simulink library "mbd_s32k_examples"  (Simulink 9.0)
settings: Solver=FixedStepDiscrete  StartTime=0.0  StopTime=10.0  FixedStep=0.1  RelTol=1e-3  EnableMultiTasking=on
InitFcn:
  | mbd_s32k14_consistency_checks(bdroot(gcs));
(part 1 of 3)
settings Model: Creator=NXP MBDT Team  LastModifiedBy=nxa14941

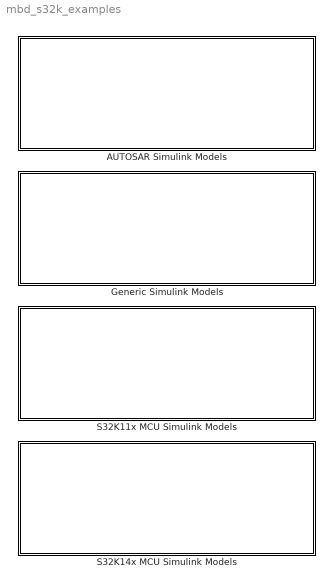
== system mbd_s32k_examples ==
  AUTOSAR Simulink Models : Subsystem
      mask Display: disp('AUTOSAR CLASSIC\n\nGenerate & Verify AUTOSAR Application Layer\non S32K1xx MCUs');
  Generic Simulink Models : Subsystem
      mask Display: disp('SIL - PIL - EXT MODE\n\nPROFILER - FREEMASTER - APPS\n\nGenerate & Verify Embedded Coder Code Generation\n on S32K1xx MCUs');
  S32K11x MCU Simulink Models : Subsystem
      mask Display: disp('S32K116, S32K118\nARM Cortex M0+\n\nCore, Systems, Peripherals, Utilities, AMMCLIB');
  S32K14x MCU Simulink Models : Subsystem
      mask Display: disp('S32K142, S32K144, S32K146, S32K148\nARM Cortex M4F\n\nCore, Systems, Peripherals, Utilities, AMMCLIB');

== system mbd_s32k_examples/AUTOSAR Simulink Models ==
  note: DISCLAIMER: All examples are distributed under the NXP Tools License Agreement Terms & Conditions
      | that can be found in LA_OPT_NXP_Software_License.htm
  note: AUTOSAR CLASSIC
      | Modelling, Verification and Validation
      | of Simulink Models on S32K1xx MCU
  "PIL " : Subsystem
      mask Display: disp('PIL\n(processor-in-the-loop)')

== system mbd_s32k_examples/Generic Simulink Models ==
  note: DISCLAIMER: All examples are distributed under the NXP Tools License Agreement Terms & Conditions that can be found in LA_OPT_NXP_Software_License.htm
  note: Modelling, Verification and Validation
      | of Simulink Models on S32K1xx MCU
  note: S32K1xx Applications
  External Mode : Subsystem
      mask Display: disp('EXTERNAL MODE')
  Miscellaneous Applications : Subsystem
      mask Display: disp('MISCELLANEOUS')
  "PIL " : Subsystem
      mask Display: disp('PIL\n(processor-in-the-loop)')
  SIL : Subsystem
      mask Display: disp('SIL\n(software-in-the-loop)')
  Utilities : Subsystem
      mask Display: disp('UTILITIES\nREGISTER ACCESS')

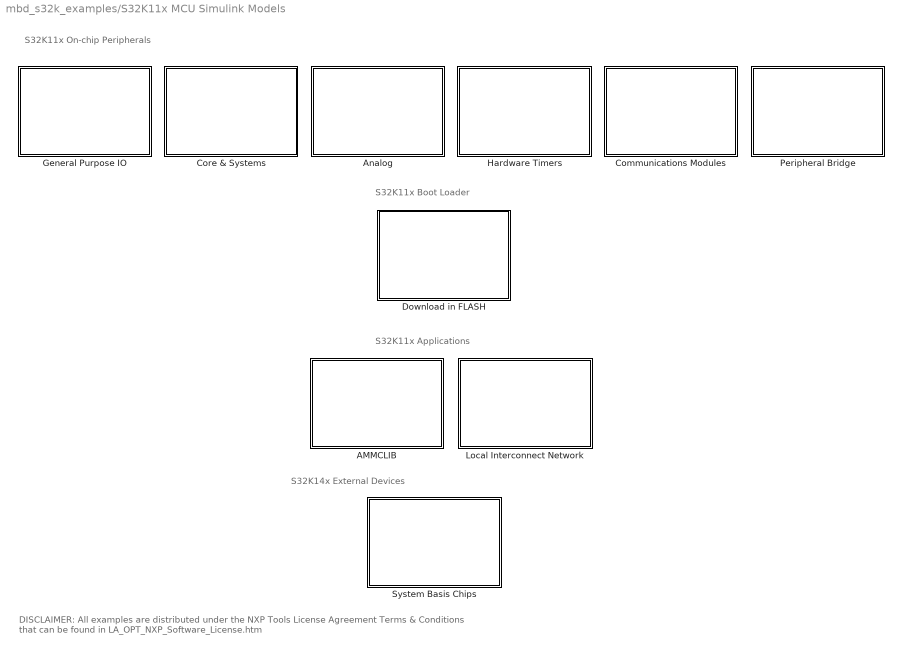
== system mbd_s32k_examples/S32K11x MCU Simulink Models ==
  note: S32K11x Boot Loader
  note: S32K11x On-chip Peripherals
  note: DISCLAIMER: All examples are distributed under the NXP Tools License Agreement Terms & Conditions that can be found in LA_OPT_NXP_Software_License.htm
  note: S32K11x Applications
  note: S32K14x External Devices
  AMMCLIB : Subsystem
      mask Display: disp('Automotive\nMath and Motor\nControl Library')
  Analog : Subsystem
      mask Display: disp('ADC\nCMP')
  Communications Modules : Subsystem
      mask Display: disp('UART\nSPI\nI2C\nFlexCAN\nFlexIO')
  Core & Systems : Subsystem
      mask Display: disp('PMC\nWDOG\nRTC\nEDMA\nLPTMR')
  Download in FLASH : Subsystem
      mask Display: disp('FLASH')
  General Purpose IO : Subsystem
      mask Display: disp('GPIO')
  Hardware Timers : Subsystem
      mask Display: disp('PDB\nFTM\nLPIT')
  Local Interconnect Network : Subsystem
      mask Display: disp('LIN')
  Peripheral Bridge : Subsystem
      mask Display: disp('MEMORIES\nREGISTERS')
  System Basis Chips : Subsystem
      mask Display: disp('SBC')

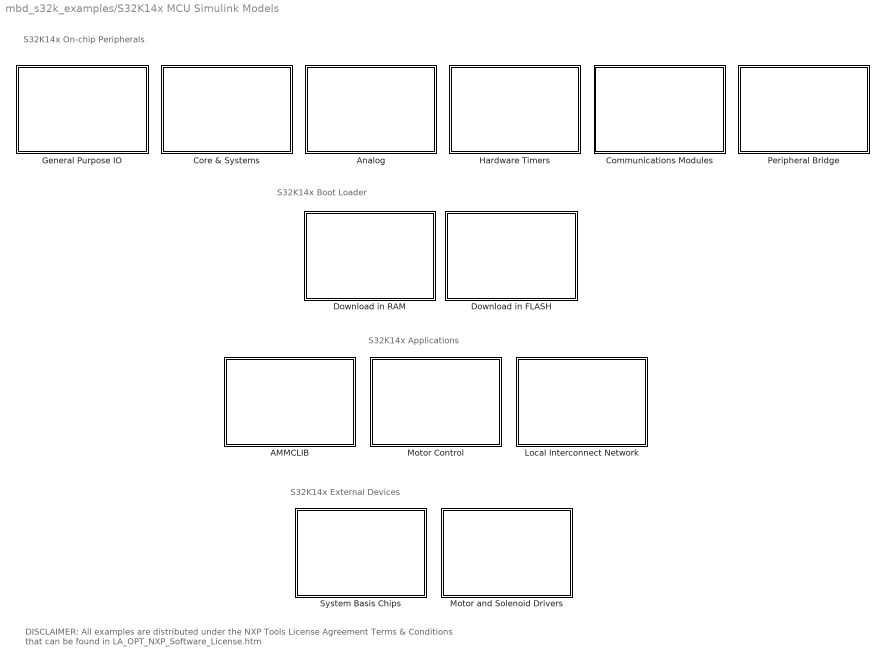
== system mbd_s32k_examples/S32K14x MCU Simulink Models ==
  note: S32K14x Boot Loader
  note: S32K14x External Devices
  note: DISCLAIMER: All examples are distributed under the NXP Tools License Agreement Terms & Conditions that can be found in LA_OPT_NXP_Software_License.htm
  note: S32K14x On-chip Peripherals
  note: S32K14x Applications
  AMMCLIB : Subsystem
      mask Display: disp('Automotive\nMath and Motor\nControl Library')
  Analog : Subsystem
      mask Display: disp('ADC\nCMP')
  Communications Modules : Subsystem
      mask Display: disp('UART\nSPI\nI2C\nFlexCAN\nFlexIO')
  Core & Systems : Subsystem
      mask Display: disp('PMC\nCSEC\nWDOG\nRTC\nEDMA\nLPTMR')
  Download in FLASH : Subsystem
      mask Display: disp('FLASH')
  Download in RAM : Subsystem
      mask Display: disp('RAM')
  General Purpose IO : Subsystem
      mask Display: disp('GPIO')
  Hardware Timers : Subsystem
      mask Display: disp('PDB\nFTM\nLPIT')
  Local Interconnect Network : Subsystem
      mask Display: disp('LIN')
  Motor Control : Subsystem
      mask Display: disp('MC')
  Motor and Solenoid Drivers : Subsystem
      mask Display: disp('TPP')
  Peripheral Bridge : Subsystem
      mask Display: disp('MEMORIES\nREGISTERS')
  System Basis Chips : Subsystem
      mask Display: disp('SBC')

== system mbd_s32k_examples/AUTOSAR Simulink Models/PIL  ==
  note: Note: PIL examples need a S32K1xx EVB to execute part of the generated code and a UART connection for getting the data out of the target. Make sure the UART port is configured correctly
  PIL_AS_Intergrator : Subsystem  mask{A=[]}
      mask prompts: A "Needed to invoke OpenFcn from the browser:"
      settings: OpenFcn=sfundemo_open('autosar_integrator_top_PIL')
      mask Display: disp('AUTOSAR PIL\nSimple Integrator');
  PIL_AS_Multiple_Runnables : Subsystem  mask{A=[]}
      mask prompts: A "Needed to invoke OpenFcn from the browser:"
      settings: OpenFcn=sfundemo_open('autosar_multirunnables_top_PIL')
      mask Display: disp('AUTOSAR PIL\nMultiple Runnables');
  PIL_AS_Throttle_Control : Subsystem  mask{A=[]}
      mask prompts: A "Needed to invoke OpenFcn from the browser:"
      settings: OpenFcn=sfundemo_open('mbdt_autosar_system_top')
      mask Display: disp('AUTOSAR PIL\nThrottle Control Example');

== system mbd_s32k_examples/Generic Simulink Models/External Mode ==
  External_Mode : Subsystem  mask{A=[]}
      mask prompts: A "Needed to invoke OpenFcn from the browser:"
      settings: OpenFcn=sfundemo_open('extmode_s32k1xx')
      mask Display: disp('EXTERNAL MODE\n Control Gauge in Simulink');

== system mbd_s32k_examples/Generic Simulink Models/Miscellaneous Applications ==
  Incremental Encoder : Subsystem  mask{A=[]}
      mask prompts: A "Needed to invoke OpenFcn from the browser:"
      settings: OpenFcn=sfundemo_open('ftm_incremental_encoder_s32k1xx')
      mask Display: disp('Incremental Encoder');

== system mbd_s32k_examples/Generic Simulink Models/PIL  ==
  note: Note: PIL examples need a S32K1xx EVB to execute part of the generated code and a UART connection for getting the data out of the target. Make sure the UART port is configured correctly
  PIL_AMMCLIB : Subsystem  mask{A=[]}
      mask prompts: A "Needed to invoke OpenFcn from the browser:"
      settings: OpenFcn=sfundemo_open('sim_pil_top_AMMCLIB_s32k1xx')
      mask Display: disp('AMMCLIB\n Sinusoidal signal generation');
  PIL_BLDC_Logic_Sequence : Subsystem  mask{A=[]}
      mask prompts: A "Needed to invoke OpenFcn from the browser:"
      settings: OpenFcn=sfundemo_open('sim_pil_top_BLDC_Commutation_s32k1xx')
      mask Display: disp('BLDC COMMUTATION\n Trapezoidal sequence commands\nand\nPWM signals output');
  PIL_RT_IO_STREAM : Subsystem  mask{A=[]}
      mask prompts: A "Needed to invoke OpenFcn from the browser:"
      settings: OpenFcn=sfundemo_open('mbd_s32k_rtiostreamtest')
      mask Display: disp('PIL TEST\nRT IO STREAM TEST');

== system mbd_s32k_examples/Generic Simulink Models/SIL ==
  SIL_AMMCLIB : Subsystem  mask{A=[]}
      mask prompts: A "Needed to invoke OpenFcn from the browser:"
      settings: OpenFcn=sfundemo_open('sim_sil_top_AMMCLIB_s32k1xx')
      mask Display: disp('AMMCLIB\n Sinusoidal signal generation');
  SIL_BLDC_Logic_Sequence : Subsystem  mask{A=[]}
      mask prompts: A "Needed to invoke OpenFcn from the browser:"
      settings: OpenFcn=sfundemo_open('sim_sil_top_BLDC_Commutation_s32k1xx')
      mask Display: disp('BLDC COMMUTATION\n Trapezoidal sequence commands\nand\nPWM signals output');
  SIL_Trapezoidal_Commutation : Subsystem  mask{A=[]}
      mask prompts: A "Needed to invoke OpenFcn from the browser:"
      settings: OpenFcn=sfundemo_open('sim_sil_top_TrapezoidalCommutation_s32k1xx')
      mask Display: disp('Trapezoidal\nCommutation');

== system mbd_s32k_examples/Generic Simulink Models/Utilities ==
  Custom_Initialization : Subsystem  mask{A=[]}
      mask prompts: A "Needed to invoke OpenFcn from the browser:"
      settings: OpenFcn=sfundemo_open('custom_init_s32k1xx')
      mask Display: disp('Custom Initialization\nCall custom code before\nat Simulink Initialize Fct');
  FreeMASTER_ISR_over_CAN : Subsystem  mask{A=[]}
      mask prompts: A "Needed to invoke OpenFcn from the browser:"
      settings: OpenFcn=sfundemo_open('fm_can_s32k1xx')
      mask Display: disp('FreeMASTER\n Data Visualization\nOver CAN');
  FreeMaster_ISR_over_UART : Subsystem  mask{A=[]}
      mask prompts: A "Needed to invoke OpenFcn from the browser:"
      settings: OpenFcn=sfundemo_open('fm_s32k1xx')
      mask Display: disp('FreeMASTER\nRECORDER and SCOPE\nInterrupt Based\nOver UART');
  FreeMaster_Polling_over_UART : Subsystem  mask{A=[]}
      mask prompts: A "Needed to invoke OpenFcn from the browser:"
      settings: OpenFcn=sfundemo_open('fm_polling_s32k1xx')
      mask Display: disp('FreeMASTER\n Polling Based\nOver UART');
  Profile_Application : Subsystem  mask{A=[]}
      mask prompts: A "Needed to invoke OpenFcn from the browser:"
      settings: OpenFcn=sfundemo_open('profiler_s32k1xx')
      mask Display: disp('PROFILER\nMeasure \nExecution Cycles');

== system mbd_s32k_examples/S32K11x MCU Simulink Models/AMMCLIB ==
  AMCLIB : Subsystem
      mask Display: disp('Advanced Motor Control Library\n\nBackEMF Observer,\n Tracking Observer,\n Speed and Current Loops');
  GDFLIB : Subsystem
      mask Display: disp('General Digital Filters Library\n\nFIR, IIR1, IIR2, Moving Average');
  GFLIB : Subsystem
      mask Display: disp('General Function Library\n\nSIN, ASIN, COS, ACOS, TAN, ATAN,\nLUT, LOG, Ramp, Hysteresis, Limit,\nPIp and PIr controllers');
  GMCLIB : Subsystem
      mask Display: disp('General Motor Control Library\n\nPark/Clark Direct&Inverse transformations,\n Space Vector Modulation,\n PMSM Decoupling,\n DC Bus Ripple Elimination');
  MLIB : Subsystem
      mask Display: disp('Mathematical Library\n\nABS, ADD, SUB, DIV, MUL, MAC,\nShifting, F16/F32/FLT Conversion');

== system mbd_s32k_examples/S32K11x MCU Simulink Models/Analog ==
  ADC_Potentiometer : Subsystem  mask{A=[]}
      mask prompts: A "Needed to invoke OpenFcn from the browser:"
      settings: OpenFcn=sfundemo_open('adc_software_trigger_s32k11x')
      mask Display: disp('ADC\nRead values from\npotentiometer');
  ADC_Software_Triggered : Subsystem  mask{A=[]}
      mask prompts: A "Needed to invoke OpenFcn from the browser:"
      settings: OpenFcn=sfundemo_open('adc_isr_s32k11x')
      mask Display: disp('ADC\nISR');
  CMP_IO_Triggering : Subsystem  mask{A=[]}
      mask prompts: A "Needed to invoke OpenFcn from the browser:"
      settings: OpenFcn=sfundemo_open('cmp_s32k11x')
      mask Display: disp('CMP\nCompare signals');
  FTM_PDB_ADC_Sync_Chaining : Subsystem  mask{A=[]}
      mask prompts: A "Needed to invoke OpenFcn from the browser:"
      settings: OpenFcn=sfundemo_open('ftm_pdb_adc_chaining_s32k11x')
      mask Display: disp('FTM-PDB-ADC\nChaining');

== system mbd_s32k_examples/S32K11x MCU Simulink Models/Communications Modules ==
  CAN : Subsystem
      mask Display: disp('FlexCAN')
  FlexIO : Subsystem
      mask Display: disp('FlexIO')
  I2C : Subsystem
      mask Display: disp('I2C')
  SPI : Subsystem
      mask Display: disp('SPI')
  Serial : Subsystem
      mask Display: disp('UART')

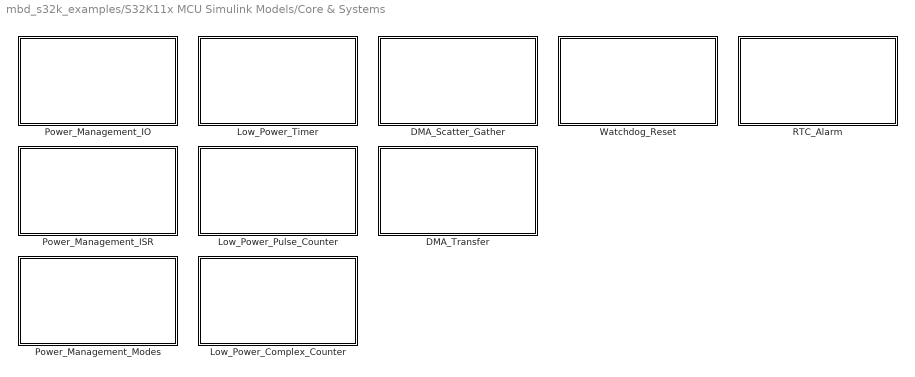
== system mbd_s32k_examples/S32K11x MCU Simulink Models/Core & Systems ==
  DMA_Scatter_Gather : Subsystem  mask{A=[]}
      mask prompts: A "Needed to invoke OpenFcn from the browser:"
      settings: OpenFcn=sfundemo_open('edma_scatter_gather_transfer_s32k11x')
      mask Display: disp('EDMA\n Scatter Gather Transfer');
  DMA_Transfer : Subsystem  mask{A=[]}
      mask prompts: A "Needed to invoke OpenFcn from the browser:"
      settings: OpenFcn=sfundemo_open('edma_simple_single_block_transfer_s32k11x')
      mask Display: disp('EDMA\n Simple Single Transfer');
  Low_Power_Complex_Counter : Subsystem  mask{A=[]}
      mask prompts: A "Needed to invoke OpenFcn from the browser:"
      settings: OpenFcn=sfundemo_open('lptmr_complex_time_counter_s32k11x')
      mask Display: disp('LPTMR\n Complex Time Counter');
  Low_Power_Pulse_Counter : Subsystem  mask{A=[]}
      mask prompts: A "Needed to invoke OpenFcn from the browser:"
      settings: OpenFcn=sfundemo_open('lptmr_pulse_counter_s32k11x')
      mask Display: disp('LPTMR\n Pulse Counter');
  Low_Power_Timer : Subsystem  mask{A=[]}
      mask prompts: A "Needed to invoke OpenFcn from the browser:"
      settings: OpenFcn=sfundemo_open('lptmr_time_counter_s32k11x')
      mask Display: disp('LPTMR\n Time Counter');
  Power_Management_IO : Subsystem  mask{A=[]}
      mask prompts: A "Needed to invoke OpenFcn from the browser:"
      settings: OpenFcn=sfundemo_open('pmc_gpio_s32k11x')
      mask Display: disp('PMC\nPower modes via GPIO');
  Power_Management_ISR : Subsystem  mask{A=[]}
      mask prompts: A "Needed to invoke OpenFcn from the browser:"
      settings: OpenFcn=sfundemo_open('pmc_callbacks_s32k11x')
      mask Display: disp('PMC\nPower modes Callbacks\n via GPIO');
  Power_Management_Modes : Subsystem  mask{A=[]}
      mask prompts: A "Needed to invoke OpenFcn from the browser:"
      settings: OpenFcn=sfundemo_open('pmc_vlpr_s32k11x')
      mask Display: disp('PMC\n Example Very Low Power Run');
  RTC_Alarm : Subsystem  mask{A=[]}
      mask prompts: A "Needed to invoke OpenFcn from the browser:"
      settings: OpenFcn=sfundemo_open('rtc_s32k11x')
      mask Display: disp('RTC');
  Watchdog_Reset : Subsystem  mask{A=[]}
      mask prompts: A "Needed to invoke OpenFcn from the browser:"
      settings: OpenFcn=sfundemo_open('wdog_s32k11x')
      mask Display: disp('WDOG');

== system mbd_s32k_examples/S32K11x MCU Simulink Models/Download in FLASH ==
  FLASH_BAM_S32K116 : Subsystem  mask{A=[]}
      mask prompts: A "Needed to invoke OpenFcn from the browser:"
      settings: OpenFcn=sfundemo_open('flash_bam_download_s32k116')
      mask Display: disp('S32K116\nDownload in Flash');
  FLASH_BAM_S32K118 : Subsystem  mask{A=[]}
      mask prompts: A "Needed to invoke OpenFcn from the browser:"
      settings: OpenFcn=sfundemo_open('flash_bam_download_s32k118')
      mask Display: disp('S32K118\nDownload in Flash');

== system mbd_s32k_examples/S32K11x MCU Simulink Models/General Purpose IO ==
  GPIO_ISR : Subsystem  mask{A=[]}
      mask prompts: A "Needed to invoke OpenFcn from the browser:"
      settings: OpenFcn=sfundemo_open('gpio_isr_control_s32k11x')
      mask Display: disp('GPIO\nISR Control');
  GPIO_S32K11xEVB : Subsystem  mask{A=[]}
      mask prompts: A "Needed to invoke OpenFcn from the browser:"
      settings: OpenFcn=sfundemo_open('gpio_s32k11x')
      mask Display: disp('GPIO on S32K11x\nLED & Buttons');

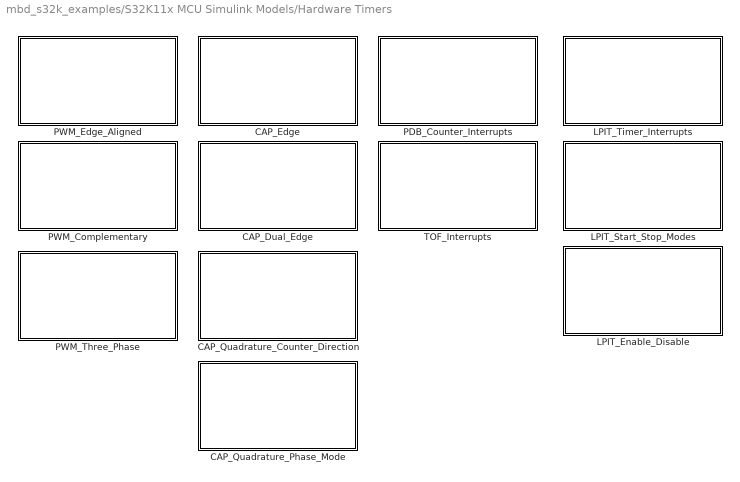
== system mbd_s32k_examples/S32K11x MCU Simulink Models/Hardware Timers ==
  CAP_Dual_Edge : Subsystem  mask{A=[]}
      mask prompts: A "Needed to invoke OpenFcn from the browser:"
      settings: OpenFcn=sfundemo_open('ftm_dual_edge_s32k11x')
      mask Display: disp('FTM\nDual Edge-Capture');
  CAP_Edge : Subsystem  mask{A=[]}
      mask prompts: A "Needed to invoke OpenFcn from the browser:"
      settings: OpenFcn=sfundemo_open('ftm_input_capture_s32k11x')
      mask Display: disp('FTM\nEdge-Capture');
  CAP_Quadrature_Counter_Direction : Subsystem  mask{A=[]}
      mask prompts: A "Needed to invoke OpenFcn from the browser:"
      settings: OpenFcn=sfundemo_open('ftm_qd_counter_s32k11x')
      mask Display: disp('FTM\nQuadrature-Capture\nCounter & Direction');
  CAP_Quadrature_Phase_Mode : Subsystem  mask{A=[]}
      mask prompts: A "Needed to invoke OpenFcn from the browser:"
      settings: OpenFcn=sfundemo_open('ftm_qd_phase_s32k11x')
      mask Display: disp('FTM\nQuadrature-Capture\nPhase Mode');
  LPIT_Enable_Disable : Subsystem  mask{A=[]}
      mask prompts: A "Needed to invoke OpenFcn from the browser:"
      settings: OpenFcn=sfundemo_open('lpit_s32k11x_enable_disable')
      mask Display: disp('LPIT\nEnable Disable');
  LPIT_Start_Stop_Modes : Subsystem  mask{A=[]}
      mask prompts: A "Needed to invoke OpenFcn from the browser:"
      settings: OpenFcn=sfundemo_open('lpit_s32k11x_start_stop')
      mask Display: disp('LPIT\nStart Stop');
  LPIT_Timer_Interrupts : Subsystem  mask{A=[]}
      mask prompts: A "Needed to invoke OpenFcn from the browser:"
      settings: OpenFcn=sfundemo_open('lpit_s32k11x')
      mask Display: disp('LPIT\nTimer interrupts');
  PDB_Counter_Interrupts : Subsystem  mask{A=[]}
      mask prompts: A "Needed to invoke OpenFcn from the browser:"
      settings: OpenFcn=sfundemo_open('pdb_s32k11x')
      mask Display: disp('PDB\nTimer interrupts');
  PWM_Complementary : Subsystem  mask{A=[]}
      mask prompts: A "Needed to invoke OpenFcn from the browser:"
      settings: OpenFcn=sfundemo_open('ftm_complementary_pwm_s32k11x')
      mask Display: disp('FTM\nComplementary\nPWM generation');
  PWM_Edge_Aligned : Subsystem  mask{A=[]}
      mask prompts: A "Needed to invoke OpenFcn from the browser:"
      settings: OpenFcn=sfundemo_open('ftm_independent_pwm_s32k11x')
      mask Display: disp('FTM\nEdge-Aligned vs\nCenter-Aligned\nPWM generation');
  PWM_Three_Phase : Subsystem  mask{A=[]}
      mask prompts: A "Needed to invoke OpenFcn from the browser:"
      settings: OpenFcn=sfundemo_open('ftm_three_phase_pwm_s32k11x')
      mask Display: disp('FTM\n3-Phase\nPWM generation\nCobine Mode');
  TOF_Interrupts : Subsystem  mask{A=[]}
      mask prompts: A "Needed to invoke OpenFcn from the browser:"
      settings: OpenFcn=sfundemo_open('ftm_tof_s32k11x')
      mask Display: disp('TOF\nTimer Overflow');

== system mbd_s32k_examples/S32K11x MCU Simulink Models/Local Interconnect Network ==
  "LIN Master " : Subsystem  mask{A=[]}
      mask prompts: A "Needed to invoke OpenFcn from the browser:"
      settings: OpenFcn=sfundemo_open('lin_master_s32k11x')
      mask Display: disp('LIN MASTER');
  LIN Slave : Subsystem  mask{A=[]}
      mask prompts: A "Needed to invoke OpenFcn from the browser:"
      settings: OpenFcn=sfundemo_open('lin_slave_s32k11x')
      mask Display: disp('LIN Slave');

== system mbd_s32k_examples/S32K11x MCU Simulink Models/Peripheral Bridge ==
  Memory_Access_RW : Subsystem  mask{A=[]}
      mask prompts: A "Needed to invoke OpenFcn from the browser:"
      settings: OpenFcn=sfundemo_open('memory_s32k11x')
      mask Display: disp('MEMORY');
  Register_Access_RW : Subsystem  mask{A=[]}
      mask prompts: A "Needed to invoke OpenFcn from the browser:"
      settings: OpenFcn=sfundemo_open('rw_registers_s32k11x')
      mask Display: disp('REGISTER');

== system mbd_s32k_examples/S32K11x MCU Simulink Models/System Basis Chips ==
  SBC_RW_Registers : Subsystem  mask{A=[]}
      mask prompts: A "Needed to invoke OpenFcn from the browser:"
      settings: OpenFcn=sfundemo_open('sbc_uja1169_rw_reg_s32k11x')
      mask Display: disp('UJA 1169\nRead/Write Registers');
  UJA1169_Control : Subsystem  mask{A=[]}
      mask prompts: A "Needed to invoke OpenFcn from the browser:"
      settings: OpenFcn=sfundemo_open('sbc_uja1169_mode_control_s32k11x')
      mask Display: disp('UJA 1169\nControl Modes');

== system mbd_s32k_examples/S32K14x MCU Simulink Models/AMMCLIB ==
  AMCLIB : Subsystem
      mask Display: disp('Advanced Motor Control Library\n\nBackEMF Observer,\n Tracking Observer,\n Speed and Current Loops');
  GDFLIB : Subsystem
      mask Display: disp('General Digital Filters Library\n\nFIR, IIR1, IIR2, Moving Average');
  GFLIB : Subsystem
      mask Display: disp('General Function Library\n\nSIN, ASIN, COS, ACOS, TAN, ATAN,\nLUT, LOG, Ramp, Hysteresis, Limit,\nPIp and PIr controllers');
  GMCLIB : Subsystem
      mask Display: disp('General Motor Control Library\n\nPark/Clark Direct&Inverse transformations,\n Space Vector Modulation,\n PMSM Decoupling,\n DC Bus Ripple Elimination');
  MLIB : Subsystem
      mask Display: disp('Mathematical Library\n\nABS, ADD, SUB, DIV, MUL, MAC,\nShifting, F16/F32/FLT Conversion');

== system mbd_s32k_examples/S32K14x MCU Simulink Models/Analog ==
  ADC_Hardware_Triggered : Subsystem  mask{A=[]}
      mask prompts: A "Needed to invoke OpenFcn from the browser:"
      settings: OpenFcn=sfundemo_open('adc_pdb_trigger_s32k14x')
      mask Display: disp('ADC\nConversion based on\nharware interrupts');
  ADC_Potentiometer : Subsystem  mask{A=[]}
      mask prompts: A "Needed to invoke OpenFcn from the browser:"
      settings: OpenFcn=sfundemo_open('adc_software_trigger_s32k14x')
      mask Display: disp('ADC\nRead values from\npotentiometer');
  ADC_Software_Triggered : Subsystem  mask{A=[]}
      mask prompts: A "Needed to invoke OpenFcn from the browser:"
      settings: OpenFcn=sfundemo_open('adc_isr_s32k14x')
      mask Display: disp('ADC\nISR');
  CMP_IO_Triggering : Subsystem  mask{A=[]}
      mask prompts: A "Needed to invoke OpenFcn from the browser:"
      settings: OpenFcn=sfundemo_open('cmp_s32k14x')
      mask Display: disp('CMP\nCompare signals');
  FTM_PDB_ADC_Sync_Chaining : Subsystem  mask{A=[]}
      mask prompts: A "Needed to invoke OpenFcn from the browser:"
      settings: OpenFcn=sfundemo_open('ftm_pdb_adc_chaining_s32k14x')
      mask Display: disp('FTM-PDB-ADC\nChaining');

== system mbd_s32k_examples/S32K14x MCU Simulink Models/Communications Modules ==
  CAN : Subsystem
      mask Display: disp('FlexCAN')
  FlexIO : Subsystem
      mask Display: disp('FlexIO')
  I2C : Subsystem
      mask Display: disp('I2C')
  SPI : Subsystem
      mask Display: disp('SPI')
  Serial : Subsystem
      mask Display: disp('UART')

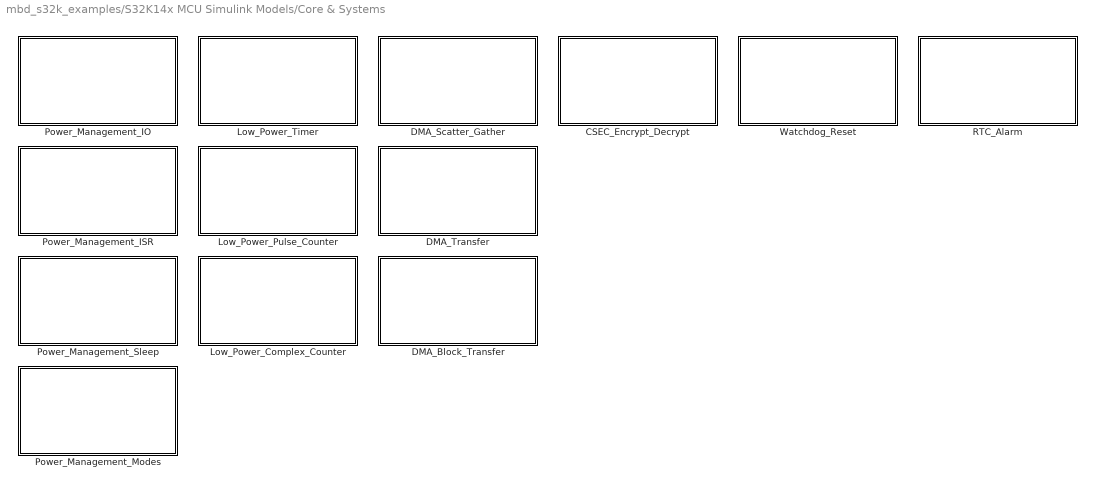
== system mbd_s32k_examples/S32K14x MCU Simulink Models/Core & Systems ==
  CSEC_Encrypt_Decrypt : Subsystem  mask{A=[]}
      mask prompts: A "Needed to invoke OpenFcn from the browser:"
      settings: OpenFcn=sfundemo_open('csec_keyconfig_s32k14x')
      mask Display: disp('CSEC');
  DMA_Block_Transfer : Subsystem  mask{A=[]}
      mask prompts: A "Needed to invoke OpenFcn from the browser:"
      settings: OpenFcn=sfundemo_open('edma_single_block_transfer_profiling_s32k14x')
      mask Display: disp('EDMA\n Single Block Transfer Profiling');
  DMA_Scatter_Gather : Subsystem  mask{A=[]}
      mask prompts: A "Needed to invoke OpenFcn from the browser:"
      settings: OpenFcn=sfundemo_open('edma_scatter_gather_transfer_s32k14x')
      mask Display: disp('EDMA\n Scatter Gather Transfer');
  DMA_Transfer : Subsystem  mask{A=[]}
      mask prompts: A "Needed to invoke OpenFcn from the browser:"
      settings: OpenFcn=sfundemo_open('edma_simple_single_block_transfer_s32k14x')
      mask Display: disp('EDMA\n Simple Single Transfer');
  Low_Power_Complex_Counter : Subsystem  mask{A=[]}
      mask prompts: A "Needed to invoke OpenFcn from the browser:"
      settings: OpenFcn=sfundemo_open('lptmr_complex_time_counter_s32k14x')
      mask Display: disp('LPTMR\n Complex Time Counter');
  Low_Power_Pulse_Counter : Subsystem  mask{A=[]}
      mask prompts: A "Needed to invoke OpenFcn from the browser:"
      settings: OpenFcn=sfundemo_open('lptmr_pulse_counter_s32k14x')
      mask Display: disp('LPTMR\n Pulse Counter');
  Low_Power_Timer : Subsystem  mask{A=[]}
      mask prompts: A "Needed to invoke OpenFcn from the browser:"
      settings: OpenFcn=sfundemo_open('lptmr_time_counter_s32k14x')
      mask Display: disp('LPTMR\n Time Counter');
  Power_Management_IO : Subsystem  mask{A=[]}
      mask prompts: A "Needed to invoke OpenFcn from the browser:"
      settings: OpenFcn=sfundemo_open('pmc_gpio_s32k14x')
      mask Display: disp('PMC\nPower modes via GPIO');
  Power_Management_ISR : Subsystem  mask{A=[]}
      mask prompts: A "Needed to invoke OpenFcn from the browser:"
      settings: OpenFcn=sfundemo_open('pmc_callbacks_s32k14x')
      mask Display: disp('PMC\nPower modes Callbacks\n via GPIO');
  Power_Management_Modes : Subsystem  mask{A=[]}
      mask prompts: A "Needed to invoke OpenFcn from the browser:"
      settings: OpenFcn=sfundemo_open('pmc_vlpr_s32k14x')
      mask Display: disp('PMC\n Example Very Low Power Run');
  Power_Management_Sleep : Subsystem  mask{A=[]}
      mask prompts: A "Needed to invoke OpenFcn from the browser:"
      settings: OpenFcn=sfundemo_open('pmc_sleep_on_exit_s32k14x')
      mask Display: disp('PMC\nPower modes Sleep on exit\nvia GPIO');
  RTC_Alarm : Subsystem  mask{A=[]}
      mask prompts: A "Needed to invoke OpenFcn from the browser:"
      settings: OpenFcn=sfundemo_open('rtc_s32k14x')
      mask Display: disp('RTC');
  Watchdog_Reset : Subsystem  mask{A=[]}
      mask prompts: A "Needed to invoke OpenFcn from the browser:"
      settings: OpenFcn=sfundemo_open('wdog_s32k14x')
      mask Display: disp('WDOG');

== system mbd_s32k_examples/S32K14x MCU Simulink Models/Download in FLASH ==
  FLASH_BAM_S32K142 : Subsystem  mask{A=[]}
      mask prompts: A "Needed to invoke OpenFcn from the browser:"
      settings: OpenFcn=sfundemo_open('flash_bam_download_s32k142')
      mask Display: disp('S32K142\nDownload in Flash');
  FLASH_BAM_S32K144 : Subsystem  mask{A=[]}
      mask prompts: A "Needed to invoke OpenFcn from the browser:"
      settings: OpenFcn=sfundemo_open('flash_bam_download_s32k144')
      mask Display: disp('S32K144\nDownload in Flash');
  FLASH_BAM_S32K146 : Subsystem  mask{A=[]}
      mask prompts: A "Needed to invoke OpenFcn from the browser:"
      settings: OpenFcn=sfundemo_open('flash_bam_download_s32k146')
      mask Display: disp('S32K146\nDownload in Flash');
  FLASH_BAM_S32K148 : Subsystem  mask{A=[]}
      mask prompts: A "Needed to invoke OpenFcn from the browser:"
      settings: OpenFcn=sfundemo_open('flash_bam_download_s32k148')
      mask Display: disp('S32K148\nDownload in Flash');

== system mbd_s32k_examples/S32K14x MCU Simulink Models/Download in RAM ==
  RAM_BAM_S32K144 : Subsystem  mask{A=[]}
      mask prompts: A "Needed to invoke OpenFcn from the browser:"
      settings: OpenFcn=sfundemo_open('ram_bam_download_s32k144')
      mask Display: disp('S32K144\nDownload in RAM');
  RAM_BAM_S32K146 : Subsystem  mask{A=[]}
      mask prompts: A "Needed to invoke OpenFcn from the browser:"
      settings: OpenFcn=sfundemo_open('ram_bam_download_s32k146')
      mask Display: disp('S32K146\nDownload in RAM');
  RAM_BAM_S32K148 : Subsystem  mask{A=[]}
      mask prompts: A "Needed to invoke OpenFcn from the browser:"
      settings: OpenFcn=sfundemo_open('ram_bam_download_s32k148')
      mask Display: disp('S32K148\nDownload in RAM');

== system mbd_s32k_examples/S32K14x MCU Simulink Models/General Purpose IO ==
  GPIO_ISR : Subsystem  mask{A=[]}
      mask prompts: A "Needed to invoke OpenFcn from the browser:"
      settings: OpenFcn=sfundemo_open('gpio_isr_control_s32k144')
      mask Display: disp('GPIO\nISR Control');
  GPIO_S32K142EVB : Subsystem  mask{A=[]}
      mask prompts: A "Needed to invoke OpenFcn from the browser:"
      settings: OpenFcn=sfundemo_open('gpio_s32k142')
      mask Display: disp('GPIO on S32K142\nLED & Buttons');
  GPIO_S32K144EVB : Subsystem  mask{A=[]}
      mask prompts: A "Needed to invoke OpenFcn from the browser:"
      settings: OpenFcn=sfundemo_open('gpio_s32k144')
      mask Display: disp('GPIO on S32K144\nLED & Buttons');
  GPIO_S32K146EVB : Subsystem  mask{A=[]}
      mask prompts: A "Needed to invoke OpenFcn from the browser:"
      settings: OpenFcn=sfundemo_open('gpio_s32k146')
      mask Display: disp('GPIO on S32K146\nLED & Buttons');
  GPIO_S32K148EVB : Subsystem  mask{A=[]}
      mask prompts: A "Needed to invoke OpenFcn from the browser:"
      settings: OpenFcn=sfundemo_open('gpio_s32k148')
      mask Display: disp('GPIO on S32K148\nLED & Buttons');

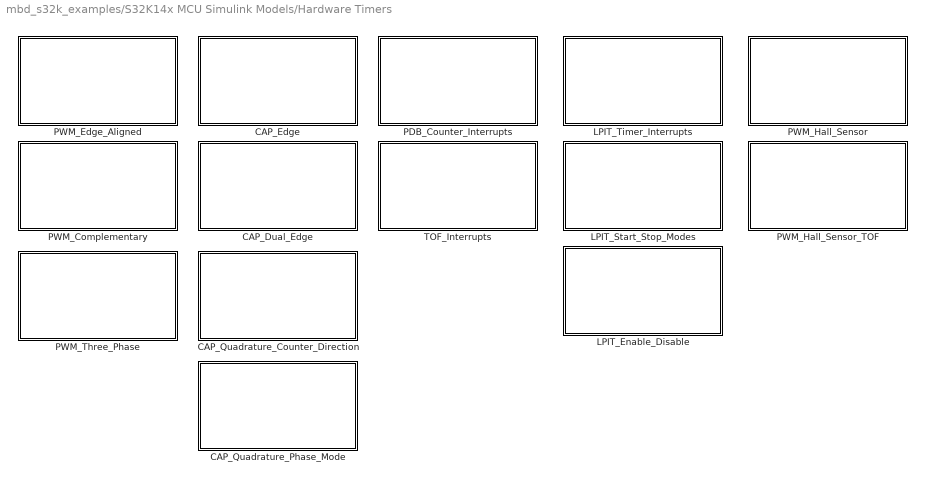
== system mbd_s32k_examples/S32K14x MCU Simulink Models/Hardware Timers ==
  CAP_Dual_Edge : Subsystem  mask{A=[]}
      mask prompts: A "Needed to invoke OpenFcn from the browser:"
      settings: OpenFcn=sfundemo_open('ftm_dual_edge_s32k14x')
      mask Display: disp('FTM\nDual Edge-Capture');
  CAP_Edge : Subsystem  mask{A=[]}
      mask prompts: A "Needed to invoke OpenFcn from the browser:"
      settings: OpenFcn=sfundemo_open('ftm_input_capture_s32k14x')
      mask Display: disp('FTM\nEdge-Capture');
  CAP_Quadrature_Counter_Direction : Subsystem  mask{A=[]}
      mask prompts: A "Needed to invoke OpenFcn from the browser:"
      settings: OpenFcn=sfundemo_open('ftm_qd_counter_s32k14x')
      mask Display: disp('FTM\nQuadrature-Capture\nCounter & Direction');
  CAP_Quadrature_Phase_Mode : Subsystem  mask{A=[]}
      mask prompts: A "Needed to invoke OpenFcn from the browser:"
      settings: OpenFcn=sfundemo_open('ftm_qd_phase_s32k14x')
      mask Display: disp('FTM\nQuadrature-Capture\nPhase Mode');
  LPIT_Enable_Disable : Subsystem  mask{A=[]}
      mask prompts: A "Needed to invoke OpenFcn from the browser:"
      settings: OpenFcn=sfundemo_open('lpit_s32k14x_enable_disable')
      mask Display: disp('LPIT\nEnable Disable');
  LPIT_Start_Stop_Modes : Subsystem  mask{A=[]}
      mask prompts: A "Needed to invoke OpenFcn from the browser:"
      settings: OpenFcn=sfundemo_open('lpit_s32k14x_start_stop')
      mask Display: disp('LPIT\nStart Stop');
  LPIT_Timer_Interrupts : Subsystem  mask{A=[]}
      mask prompts: A "Needed to invoke OpenFcn from the browser:"
      settings: OpenFcn=sfundemo_open('lpit_s32k14x')
      mask Display: disp('LPIT\nTimer interrupts');
  PDB_Counter_Interrupts : Subsystem  mask{A=[]}
      mask prompts: A "Needed to invoke OpenFcn from the browser:"
      settings: OpenFcn=sfundemo_open('pdb_s32k14x')
      mask Display: disp('PDB\nTimer interrupts');
  PWM_Complementary : Subsystem  mask{A=[]}
      mask prompts: A "Needed to invoke OpenFcn from the browser:"
      settings: OpenFcn=sfundemo_open('ftm_complementary_pwm_s32k14x')
      mask Display: disp('FTM\nComplementary\nPWM generation');
  PWM_Edge_Aligned : Subsystem  mask{A=[]}
      mask prompts: A "Needed to invoke OpenFcn from the browser:"
      settings: OpenFcn=sfundemo_open('ftm_independent_pwm_s32k14x')
      mask Display: disp('FTM\nEdge-Aligned vs\nCenter-Aligned\nPWM generation');
  PWM_Hall_Sensor : Subsystem  mask{A=[]}
      mask prompts: A "Needed to invoke OpenFcn from the browser:"
      settings: OpenFcn=sfundemo_open('ftm_hall_sensor_s32k14x')
      mask Display: disp('FTM\nHall Sensor');
  PWM_Hall_Sensor_TOF : Subsystem  mask{A=[]}
      mask prompts: A "Needed to invoke OpenFcn from the browser:"
      settings: OpenFcn=sfundemo_open('ftm_hall_sensor_tof_s32k14x')
      mask Display: disp('FTM\nHall Sensor TOF');
  PWM_Three_Phase : Subsystem  mask{A=[]}
      mask prompts: A "Needed to invoke OpenFcn from the browser:"
      settings: OpenFcn=sfundemo_open('ftm_three_phase_pwm_s32k14x')
      mask Display: disp('FTM\n3-Phase\nPWM generation\nCobine Mode');
  TOF_Interrupts : Subsystem  mask{A=[]}
      mask prompts: A "Needed to invoke OpenFcn from the browser:"
      settings: OpenFcn=sfundemo_open('ftm_tof_s32k14x')
      mask Display: disp('TOF\nTimer Overflow');

== system mbd_s32k_examples/S32K14x MCU Simulink Models/Local Interconnect Network ==
  "LIN Master " : Subsystem  mask{A=[]}
      mask prompts: A "Needed to invoke OpenFcn from the browser:"
      settings: OpenFcn=sfundemo_open('lin_master_s32k14x')
      mask Display: disp('LIN MASTER');
  LIN Slave : Subsystem  mask{A=[]}
      mask prompts: A "Needed to invoke OpenFcn from the browser:"
      settings: OpenFcn=sfundemo_open('lin_slave_s32k14x')
      mask Display: disp('LIN Slave');

== system mbd_s32k_examples/S32K14x MCU Simulink Models/Motor Control ==
  note: CAUTION: read carefully each example description and notes. Damage may occurs if the connections or supply voltage are not set properly
  note: DISCLAIMER: These Simulink models were tested on a custom setup: S32K144EVB-Q100 revX3, MotorGD revX1 and Linix Motor 45ZWN24-40-B.
      | These models implements a custom commutation table which is dependent on motor and phases/hall sensors connections order.
      |
      | Read very carefully the HW&SW Setup for each example provided.
      | All examples are distributed under the NXP Tools License Agreement Terms & Conditions that can be found in LA_OPT_NXP_Software_License.htm
  6-step commutation sequence based on Hall Sensors transitions  and PI Speed Controller : Subsystem  mask{A=[]}
      mask prompts: A "Needed to invoke OpenFcn from the browser:"
      settings: OpenFcn=sfundemo_open('BLDC_ClosedLoop_s32k144')
      mask Display: disp('BLDC: CLOSED LOOP\nSpeed Control');
  "6-step commutation sequence  based on Hall Sensors transitions " : Subsystem  mask{A=[]}
      mask prompts: A "Needed to invoke OpenFcn from the browser:"
      settings: OpenFcn=sfundemo_open('BLDC_OpenLoop_s32k144')
      mask Display: disp('BLDC: OPEN LOOP\nHall Commutation');
  Closed Loop Speed Control with FOC and Speed Estimator Based on Hall Sensors : Subsystem  mask{A=[]}
      mask prompts: A "Needed to invoke OpenFcn from the browser:"
      settings: OpenFcn=sfundemo_open('PMSM_ClosedLoop_s32k144')
      mask Display: disp('PMSM: CLOSED LOOP\nSpeed Control');
  FOC Open Loop based on V/f control method : Subsystem  mask{A=[]}
      mask prompts: A "Needed to invoke OpenFcn from the browser:"
      settings: OpenFcn=sfundemo_open('PMSM_OpenLoop_s32k144')
      mask Display: disp('PMSM: OPEN LOOP\nV/f Control');

== system mbd_s32k_examples/S32K14x MCU Simulink Models/Motor and Solenoid Drivers ==
  MC34GD3000_Configuration : Subsystem  mask{A=[]}
      mask prompts: A "Needed to invoke OpenFcn from the browser:"
      settings: OpenFcn=sfundemo_open('tpp_config_interrupt_read_write_register')
      mask Display: disp('MC34GD3000\nConfiguration');
  MC34GD3000_Functional_Mode : Subsystem  mask{A=[]}
      mask prompts: A "Needed to invoke OpenFcn from the browser:"
      settings: OpenFcn=sfundemo_open('tpp_functional_mode')
      mask Display: disp('MC34GD3000\nFunctional Mode');

== system mbd_s32k_examples/S32K14x MCU Simulink Models/Peripheral Bridge ==
  Memory_Access_RW : Subsystem  mask{A=[]}
      mask prompts: A "Needed to invoke OpenFcn from the browser:"
      settings: OpenFcn=sfundemo_open('memory_s32k14x')
      mask Display: disp('MEMORY');
  Register_Access_RW : Subsystem  mask{A=[]}
      mask prompts: A "Needed to invoke OpenFcn from the browser:"
      settings: OpenFcn=sfundemo_open('rw_registers_s32k14x')
      mask Display: disp('REGISTER');

== system mbd_s32k_examples/S32K14x MCU Simulink Models/System Basis Chips ==
  SBC_RW_Registers : Subsystem  mask{A=[]}
      mask prompts: A "Needed to invoke OpenFcn from the browser:"
      settings: OpenFcn=sfundemo_open('sbc_uja1169_write_reg_s32k14x')
      mask Display: disp('UJA 1169\nRead/Write Registers');
  "SBC_RW_Registers " : Subsystem  mask{A=[]}
      mask prompts: A "Needed to invoke OpenFcn from the browser:"
      settings: OpenFcn=sfundemo_open('sbc_uja113x_rw_reg_s32k148')
      mask Display: disp('UJA 113x\nRead/Write Registers');
  SBC_Write_Registers : Subsystem  mask{A=[]}
      mask prompts: A "Needed to invoke OpenFcn from the browser:"
      settings: OpenFcn=sfundemo_open('sbc_uja1169_rw_reg_s32k14x')
      mask Display: disp('UJA 1169\nWrite Registers');
  UJA113x_Control : Subsystem  mask{A=[]}
      mask prompts: A "Needed to invoke OpenFcn from the browser:"
      settings: OpenFcn=sfundemo_open('sbc_uja113x_mode_control_s32k148')
      mask Display: disp('UJA 113x\nControl Modes');
  UJA1169_Control : Subsystem  mask{A=[]}
      mask prompts: A "Needed to invoke OpenFcn from the browser:"
      settings: OpenFcn=sfundemo_open('sbc_uja1169_mode_control_s32k14x')
      mask Display: disp('UJA 1169\nControl Modes');

== system mbd_s32k_examples/AUTOSAR Simulink Models/PIL /PIL_AS_Intergrator ==
  Gain : Gain  SaturateOnIntegerOverflow=on  OutDataTypeStr=Inherit: Same as input  ParamDataTypeStr=Inherit: Same as input

== system mbd_s32k_examples/AUTOSAR Simulink Models/PIL /PIL_AS_Multiple_Runnables ==
  Gain : Gain  SaturateOnIntegerOverflow=on  OutDataTypeStr=Inherit: Same as input  ParamDataTypeStr=Inherit: Same as input

== system mbd_s32k_examples/AUTOSAR Simulink Models/PIL /PIL_AS_Throttle_Control ==
  Gain : Gain  SaturateOnIntegerOverflow=on  OutDataTypeStr=Inherit: Same as input  ParamDataTypeStr=Inherit: Same as input

== system mbd_s32k_examples/Generic Simulink Models/External Mode/External_Mode ==
  Gain : Gain  SaturateOnIntegerOverflow=on  OutDataTypeStr=Inherit: Same as input  ParamDataTypeStr=Inherit: Same as input

== system mbd_s32k_examples/Generic Simulink Models/Miscellaneous Applications/Incremental Encoder ==
  Gain : Gain  SaturateOnIntegerOverflow=on  OutDataTypeStr=Inherit: Same as input  ParamDataTypeStr=Inherit: Same as input

== system mbd_s32k_examples/Generic Simulink Models/PIL /PIL_AMMCLIB ==
  Gain : Gain  SaturateOnIntegerOverflow=on  OutDataTypeStr=Inherit: Same as input  ParamDataTypeStr=Inherit: Same as input

== system mbd_s32k_examples/Generic Simulink Models/PIL /PIL_BLDC_Logic_Sequence ==
  Gain : Gain  SaturateOnIntegerOverflow=on  OutDataTypeStr=Inherit: Same as input  ParamDataTypeStr=Inherit: Same as input

== system mbd_s32k_examples/Generic Simulink Models/PIL /PIL_RT_IO_STREAM ==
  Gain : Gain  SaturateOnIntegerOverflow=on  OutDataTypeStr=Inherit: Same as input  ParamDataTypeStr=Inherit: Same as input

== system mbd_s32k_examples/Generic Simulink Models/SIL/SIL_AMMCLIB ==
  Gain : Gain  SaturateOnIntegerOverflow=on  OutDataTypeStr=Inherit: Same as input  ParamDataTypeStr=Inherit: Same as input

== system mbd_s32k_examples/Generic Simulink Models/SIL/SIL_BLDC_Logic_Sequence ==
  Gain : Gain  SaturateOnIntegerOverflow=on  OutDataTypeStr=Inherit: Same as input  ParamDataTypeStr=Inherit: Same as input

== system mbd_s32k_examples/Generic Simulink Models/SIL/SIL_Trapezoidal_Commutation ==
  Gain : Gain  SaturateOnIntegerOverflow=on  OutDataTypeStr=Inherit: Same as input  ParamDataTypeStr=Inherit: Same as input

== system mbd_s32k_examples/Generic Simulink Models/Utilities/Custom_Initialization ==
  Gain : Gain  SaturateOnIntegerOverflow=on  OutDataTypeStr=Inherit: Same as input  ParamDataTypeStr=Inherit: Same as input

== system mbd_s32k_examples/Generic Simulink Models/Utilities/FreeMASTER_ISR_over_CAN ==
  Gain : Gain  SaturateOnIntegerOverflow=on  OutDataTypeStr=Inherit: Same as input  ParamDataTypeStr=Inherit: Same as input

== system mbd_s32k_examples/Generic Simulink Models/Utilities/FreeMaster_ISR_over_UART ==
  Gain : Gain  SaturateOnIntegerOverflow=on  OutDataTypeStr=Inherit: Same as input  ParamDataTypeStr=Inherit: Same as input

== system mbd_s32k_examples/Generic Simulink Models/Utilities/FreeMaster_Polling_over_UART ==
  Gain : Gain  SaturateOnIntegerOverflow=on  OutDataTypeStr=Inherit: Same as input  ParamDataTypeStr=Inherit: Same as input

== system mbd_s32k_examples/Generic Simulink Models/Utilities/Profile_Application ==
  Gain : Gain  SaturateOnIntegerOverflow=on  OutDataTypeStr=Inherit: Same as input  ParamDataTypeStr=Inherit: Same as input

== system mbd_s32k_examples/S32K11x MCU Simulink Models/AMMCLIB/AMCLIB ==
  AMCLIB_BackEMF_OBSERVER_F16 : Subsystem  mask{A=[]}
      mask prompts: A "Needed to invoke OpenFcn from the browser:"
      settings: OpenFcn=sfundemo_open('ammclib_amclib_observer_F16_s32k11x')
      mask Display: disp('OBSERVERS\nBackEMF observer and\nPosition Tracking observer\nexample for F16 datatypes');
  AMCLIB_BackEMF_OBSERVER_F32 : Subsystem  mask{A=[]}
      mask prompts: A "Needed to invoke OpenFcn from the browser:"
      settings: OpenFcn=sfundemo_open('ammclib_amclib_observer_F32_s32k11x')
      mask Display: disp('OBSERVERS\nBackEMF observer and\nPosition Tracking observer\nexample for F32 datatypes');
  AMCLIB_CURRENT_LOOP : Subsystem  mask{A=[]}
      mask prompts: A "Needed to invoke OpenFcn from the browser:"
      settings: OpenFcn=sfundemo_open('ammclib_amclib_current_loop_s32k11x')
      mask Display: disp('CURRENT LOOP\nCurrent Loop FOC\n for F16/F32 datatypes');
  AMCLIB_FW : Subsystem  mask{A=[]}
      mask prompts: A "Needed to invoke OpenFcn from the browser:"
      settings: OpenFcn=sfundemo_open('ammclib_amclib_field_weakening_s32k11x')
      mask Display: disp('FW\nField-Weakening Algorithm\non PMSM examples\n for F16/F32 datatypes');
  AMCLIB_SPEED_LOOP : Subsystem  mask{A=[]}
      mask prompts: A "Needed to invoke OpenFcn from the browser:"
      settings: OpenFcn=sfundemo_open('ammclib_amclib_speed_loop_s32k11x')
      mask Display: disp('SPEED LOOP\nSpeed Loop FOC\n for F16/F32 datatypes');
  AMCLIB_SPEED_LOOP_with_FW : Subsystem  mask{A=[]}
      mask prompts: A "Needed to invoke OpenFcn from the browser:"
      settings: OpenFcn=sfundemo_open('ammclib_amclib_FW_speed_loop_s32k11x')
      mask Display: disp('FW SPEED LOOP\nSpeed Loop with\nField Weakening examples\nfor F16/F32 datatypes');

== system mbd_s32k_examples/S32K11x MCU Simulink Models/AMMCLIB/GDFLIB ==
  GDFLIB_FIR : Subsystem  mask{A=[]}
      mask prompts: A "Needed to invoke OpenFcn from the browser:"
      settings: OpenFcn=sfundemo_open('ammclib_gdflib_fir_s32k11x')
      mask Display: disp('FIR\nFinite Impulse Response filter for\nF16/F32 datatypes');
  GDFLIB_IIR1 : Subsystem  mask{A=[]}
      mask prompts: A "Needed to invoke OpenFcn from the browser:"
      settings: OpenFcn=sfundemo_open('ammclib_gdflib_iir1_s32k11x')
      mask Display: disp('IIR1\nFirst order\nInfinite Impulse Response filter for\nF16/F32 datatypes');
  GDFLIB_IIR2 : Subsystem  mask{A=[]}
      mask prompts: A "Needed to invoke OpenFcn from the browser:"
      settings: OpenFcn=sfundemo_open('ammclib_gdflib_iir2_s32k11x')
      mask Display: disp('IIR2\nSecond order\nInfinite Impulse Response filter for\nF16/F32 datatypes');
  GDFLIB_MA : Subsystem  mask{A=[]}
      mask prompts: A "Needed to invoke OpenFcn from the browser:"
      settings: OpenFcn=sfundemo_open('ammclib_gdflib_ma_s32k11x')
      mask Display: disp('MA\nMoving Average filter for\nF16/F32 datatypes');

== system mbd_s32k_examples/S32K11x MCU Simulink Models/AMMCLIB/GFLIB ==
  GFLIB_LIMIT : Subsystem  mask{A=[]}
      mask prompts: A "Needed to invoke OpenFcn from the browser:"
      settings: OpenFcn=sfundemo_open('ammclib_gflib_limit_s32k11x')
      mask Display: disp('LIMIT\nScalar and Vector\nlimiting examples for\nF16/F32 datatypes');
  GFLIB_LUT : Subsystem  mask{A=[]}
      mask prompts: A "Needed to invoke OpenFcn from the browser:"
      settings: OpenFcn=sfundemo_open('ammclib_gflib_lut_s32k11x')
      mask Display: disp('LUT\nLook-up-Tables examples for\nF16/F32 datatypes');
  GFLIB_MISCELLANEOUS : Subsystem  mask{A=[]}
      mask prompts: A "Needed to invoke OpenFcn from the browser:"
      settings: OpenFcn=sfundemo_open('ammclib_gflib_miscellaneous_s32k11x')
      mask Display: disp('MISC\nSQRT/SIGN/INT/RAMP/HYST\n examples for\nF16/F32 datatypes');
  GFLIB_PIP : Subsystem  mask{A=[]}
      mask prompts: A "Needed to invoke OpenFcn from the browser:"
      settings: OpenFcn=sfundemo_open('ammclib_gflib_pip_s32k11x')
      mask Display: disp('PIp\nPI parallel form examples for\nF16/F32 datatypes');
  GFLIB_PIR : Subsystem  mask{A=[]}
      mask prompts: A "Needed to invoke OpenFcn from the browser:"
      settings: OpenFcn=sfundemo_open('ammclib_gflib_pir_s32k11x')
      mask Display: disp('PIr\nPI reccurent form examples for\nF16/F32 datatypes');
  GFLIB_TRIGONOMETRIC : Subsystem  mask{A=[]}
      mask prompts: A "Needed to invoke OpenFcn from the browser:"
      settings: OpenFcn=sfundemo_open('ammclib_gflib_trigonometric_s32k11x')
      mask Display: disp('TRIGONOMETRIC\nTrigonometric SIN/COS/TAN\n examples for\nF16/F32 datatypes');

== system mbd_s32k_examples/S32K11x MCU Simulink Models/AMMCLIB/GMCLIB ==
  GMCLIB_FOC_F16 : Subsystem  mask{A=[]}
      mask prompts: A "Needed to invoke OpenFcn from the browser:"
      settings: OpenFcn=sfundemo_open('ammclib_gmclib_foc_F16_s32k11x')
      mask Display: disp('FOC\nField Oriented Control\nCoordinate Transformations and\nPWM signal generation\nexample for\nF16 datatypes');
  GMCLIB_FOC_F32 : Subsystem  mask{A=[]}
      mask prompts: A "Needed to invoke OpenFcn from the browser:"
      settings: OpenFcn=sfundemo_open('ammclib_gmclib_foc_F32_s32k11x')
      mask Display: disp('FOC\nField Oriented Control\nCoordinate Transformations and\nPWM signal generation\nexample for\nF32 datatypes');

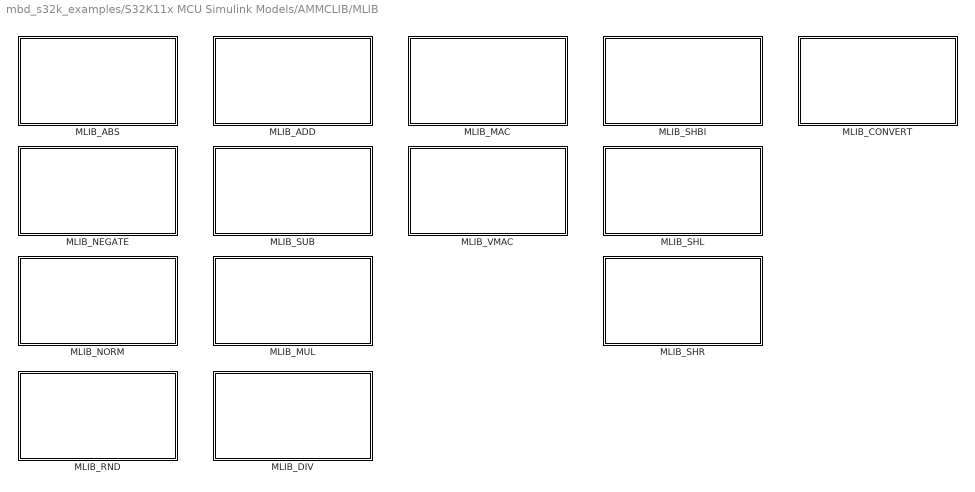
== system mbd_s32k_examples/S32K11x MCU Simulink Models/AMMCLIB/MLIB ==
  MLIB_ABS : Subsystem  mask{A=[]}
      mask prompts: A "Needed to invoke OpenFcn from the browser:"
      settings: OpenFcn=sfundemo_open('ammclib_mlib_abs_s32k11x')
      mask Display: disp('ABS\nModulo examples for\nF16/F32 datatypes');
  MLIB_ADD : Subsystem  mask{A=[]}
      mask prompts: A "Needed to invoke OpenFcn from the browser:"
      settings: OpenFcn=sfundemo_open('ammclib_mlib_add_s32k11x')
      mask Display: disp('ADD\nAddition examples for\nF16/F32 datatypes');
  MLIB_CONVERT : Subsystem  mask{A=[]}
      mask prompts: A "Needed to invoke OpenFcn from the browser:"
      settings: OpenFcn=sfundemo_open('ammclib_mlib_convert_s32k11x')
      mask Display: disp('CONVERT\nType conversions for\nF16/F32 datatypes');
  MLIB_DIV : Subsystem  mask{A=[]}
      mask prompts: A "Needed to invoke OpenFcn from the browser:"
      settings: OpenFcn=sfundemo_open('ammclib_mlib_div_s32k11x')
      mask Display: disp('DIV\nDivision examples for\nF16/F32 datatypes');
  MLIB_MAC : Subsystem  mask{A=[]}
      mask prompts: A "Needed to invoke OpenFcn from the browser:"
      settings: OpenFcn=sfundemo_open('ammclib_mlib_mac_s32k11x')
      mask Display: disp('MAC\nMultiplication with\n Addition/Substraction examples for\nF16/F32 datatypes');
  MLIB_MUL : Subsystem  mask{A=[]}
      mask prompts: A "Needed to invoke OpenFcn from the browser:"
      settings: OpenFcn=sfundemo_open('ammclib_mlib_mul_s32k11x')
      mask Display: disp('MUL\nMultiplication examples for\nF16/F32 datatypes');
  MLIB_NEGATE : Subsystem  mask{A=[]}
      mask prompts: A "Needed to invoke OpenFcn from the browser:"
      settings: OpenFcn=sfundemo_open('ammclib_mlib_neg_s32k11x')
      mask Display: disp('NEGATE\nNegate examples for\nF16/F32 datatypes');
  MLIB_NORM : Subsystem  mask{A=[]}
      mask prompts: A "Needed to invoke OpenFcn from the browser:"
      settings: OpenFcn=sfundemo_open('ammclib_mlib_norm_s32k11x')
      mask Display: disp('NORM\nNormalization examples for\nF16/F32 datatypes');
  MLIB_RND : Subsystem  mask{A=[]}
      mask prompts: A "Needed to invoke OpenFcn from the browser:"
      settings: OpenFcn=sfundemo_open('ammclib_mlib_rnd_s32k11x')
      mask Display: disp('RND\nRound examples for\nF16/F32 datatypes');
  MLIB_SHBI : Subsystem  mask{A=[]}
      mask prompts: A "Needed to invoke OpenFcn from the browser:"
      settings: OpenFcn=sfundemo_open('ammclib_mlib_shbi_s32k11x')
      mask Display: disp('SHBI\nBidirectional Shift examples for\nF16/F32 datatypes');
  MLIB_SHL : Subsystem  mask{A=[]}
      mask prompts: A "Needed to invoke OpenFcn from the browser:"
      settings: OpenFcn=sfundemo_open('ammclib_mlib_shl_s32k11x')
      mask Display: disp('SHL\nLeft Shift examples for\nF16/F32 datatypes');
  MLIB_SHR : Subsystem  mask{A=[]}
      mask prompts: A "Needed to invoke OpenFcn from the browser:"
      settings: OpenFcn=sfundemo_open('ammclib_mlib_shr_s32k11x')
      mask Display: disp('SHR\nRight Shift examples for\nF16/F32 datatypes');
  MLIB_SUB : Subsystem  mask{A=[]}
      mask prompts: A "Needed to invoke OpenFcn from the browser:"
      settings: OpenFcn=sfundemo_open('ammclib_mlib_sub_s32k11x')
      mask Display: disp('SUB\nSubstraction examples for\nF16/F32 datatypes');
  MLIB_VMAC : Subsystem  mask{A=[]}
      mask prompts: A "Needed to invoke OpenFcn from the browser:"
      settings: OpenFcn=sfundemo_open('ammclib_mlib_vmac_s32k11x')
      mask Display: disp('VMAC\nVector multiplication examples for\nF16/F32 datatypes');

== system mbd_s32k_examples/S32K11x MCU Simulink Models/Analog/ADC_Potentiometer ==
  Gain : Gain  SaturateOnIntegerOverflow=on  OutDataTypeStr=Inherit: Same as input  ParamDataTypeStr=Inherit: Same as input

== system mbd_s32k_examples/S32K11x MCU Simulink Models/Analog/ADC_Software_Triggered ==
  Gain : Gain  SaturateOnIntegerOverflow=on  OutDataTypeStr=Inherit: Same as input  ParamDataTypeStr=Inherit: Same as input

== system mbd_s32k_examples/S32K11x MCU Simulink Models/Analog/CMP_IO_Triggering ==
  Gain : Gain  SaturateOnIntegerOverflow=on  OutDataTypeStr=Inherit: Same as input  ParamDataTypeStr=Inherit: Same as input

== system mbd_s32k_examples/S32K11x MCU Simulink Models/Analog/FTM_PDB_ADC_Sync_Chaining ==
  Gain : Gain  SaturateOnIntegerOverflow=on  OutDataTypeStr=Inherit: Same as input  ParamDataTypeStr=Inherit: Same as input
